simulink model "rc_feedthrough"  (R2025b)
settings: Solver=ode2  StartTime=0.0  StopTime=inf  FixedStep=0.01  RelTol=1e-3
settings Model: Creator=ac112430  LastModifiedBy=ac124458
settings SolverCC: AlgebraicLoopSolver=TrustRegion
settings DataIOCC: ReturnWorkspaceOutputs=off
settings OptimizationCC: DefaultParameterBehavior=Inlined  DefaultUnderspecifiedDataType=single  ReuseModelBlockBuffer=off  PassReuseOutputArgsAs=Individual arguments  EfficientTunableParamExpr=on
settings DebuggingCC: ParameterPrecisionLossMsg=none  ParameterTunabilityLossMsg=error  UnconnectedInputMsg=warning  UnconnectedOutputMsg=warning  UnconnectedLineMsg=warning  ArithmeticOperatorsInVariantConditions=warning
settings HardwareCC: ProdBitPerPointer=32.0  ProdBitPerSizeT=32.0  ProdBitPerPtrDiffT=32.0  ProdLargestAtomicInteger=Long  ProdLargestAtomicFloat=Double  ProdIntDivRoundTo=Undefined  ProdWordSize=32.0  ProdLongLongMode=on  ProdHWDeviceType=ARM Compatible->ARM Cortex
settings ModelReferenceCC: EnableRefExpFcnMdlSchedulingChecks=on  ModelReferenceNumInstancesAllowed=Single  PropagateSignalLabelsOutOfModel=off
settings SFSimCC: SimUseLocalCustomCode=off  MATLABDynamicMemAlloc=off  CustomCodeUndefinedFunction=UseInterfaceOnly
settings RTWCC: SystemTargetFile=ert.tlc  GenCodeOnly=on  TemplateMakefile=ert_default_tmf  RTWUseLocalCustomCode=off  IncludeHyperlinkInReport=on  GPUComputeCapability=3.5  DLArmComputeVersion=19.05  Description=Embedded Coder
settings CodeAppCC: IgnoreCustomStorageClasses=off  MaxIdLength=63.0  StateflowObjectComments=on
settings ERTTargetCC: ERTCustomFileTemplate=example_file_process.tlc  ConvertIfToSwitch=off  SuppressUnreachableDefaultCases=off  DynamicArrayContainerType=coder::array  TargetLangStandard=C99 (ISO)  GenerateSampleERTMain=on  SupportComplex=off

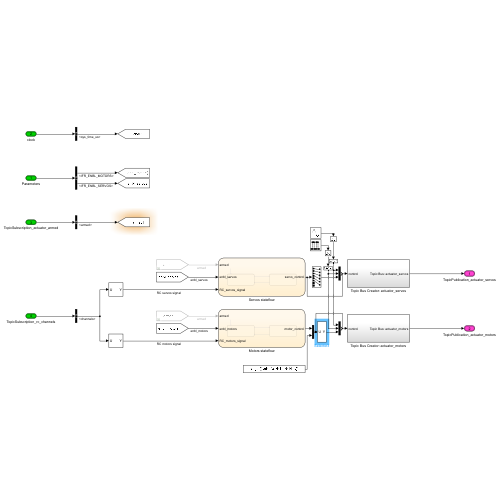
[thumbnail: Simulink's stored preview of the top-level diagram]
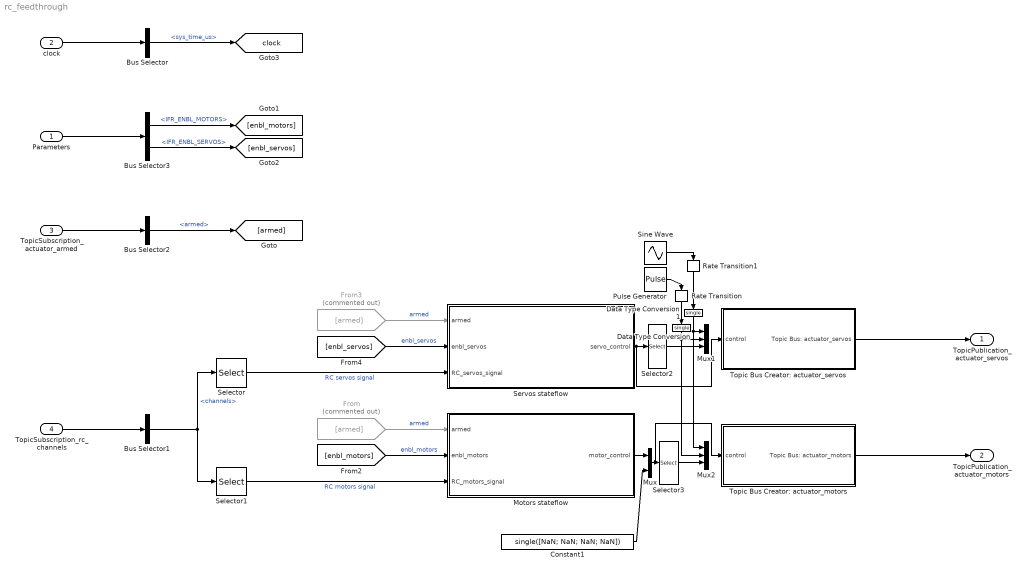
== system rc_feedthrough ==
  Parameters : Inport  OutDataTypeStr=Bus: IFRCG_Bus_Params
  clock : Inport  Port=2  OutDataTypeStr=Bus: IFRCG_Bus_CodeGenInternalClock
  TopicSubscription_actuator_armed : Inport  Port=3  OutDataTypeStr=Bus: IFRCG_Bus_Topic_ActuatorArmed
  TopicSubscription_rc_channels : Inport  Port=4  OutDataTypeStr=Bus: IFRCG_Bus_Topic_RcChannels
  Bus Selector : BusSelector  OutputSignals=sys_time_us
  Bus Selector1 : BusSelector  OutputSignals=channels
  Bus Selector2 : BusSelector  OutputSignals=armed
  Bus Selector3 : BusSelector  OutputSignals=Ifr_Feedthrough.IFR_ENBL_MOTORS,Ifr_Feedthrough.IFR_ENBL_SERVOS
  Constant1 : Constant  Value=single([NaN; NaN; NaN; NaN])  OutDataTypeStr=single
  Data Type Conversion : DataTypeConversion  OutDataTypeStr=single  SaturateOnIntegerOverflow=off  RndMeth=Floor
  Data Type Conversion1 : DataTypeConversion  OutDataTypeStr=single  SaturateOnIntegerOverflow=off  RndMeth=Floor
  From : From  Commented=on  GotoTag=armed
  From3 : From  Commented=on  GotoTag=armed
  Motors stateflow : Stateflow chart  TreatAsAtomicUnit=on
  Mux : Mux  Inputs=2
  Mux1 : Mux  Inputs=3
  Mux2 : Mux  Inputs=3
  Pulse Generator : DiscretePulseGenerator  Period=1000  PulseWidth=50  SampleTime=-1
  Rate Transition : RateTransition
  Rate Transition1 : RateTransition
  Selector : Selector  InputPortWidth=18  IndexOptions=Index vector (dialog)  Indices=[1 2 3 4 5 6 15 16]  OutputSizes=1
  Selector1 : Selector  InputPortWidth=18  IndexOptions=Index vector (dialog)  Indices=[7 8 9 10 11 12 13 14]  OutputSizes=1
  Selector2 : Selector  InputPortWidth=8  IndexOptions=Index vector (dialog)  Indices=1:6  OutputSizes=1
  Selector3 : Selector  InputPortWidth=12  IndexOptions=Index vector (dialog)  Indices=1:10  OutputSizes=1
  Servos stateflow : Stateflow chart  TreatAsAtomicUnit=on
  Sine Wave : Sin  SineType=Sample based  Samples=1000  SampleTime=0.01
  Topic Bus Creator: actuator_motors : Subsystem
  Topic Bus Creator: actuator_servos : Subsystem
  TopicPublication_actuator_servos : Outport  OutDataTypeStr=Bus: IFRCG_Bus_Topic_ActuatorServos  SampleTime=[0.01,0]  VectorParamsAs1DForOutWhenUnconnected=off
  TopicPublication_actuator_motors : Outport  Port=2  OutDataTypeStr=Bus: IFRCG_Bus_Topic_ActuatorMotors  SampleTime=[0.01,0]  VectorParamsAs1DForOutWhenUnconnected=off
  tag scope: clock=global
  wires:
  clock/1 -> Bus Selector/1
  Parameters/1 -> Bus Selector3/1
  Bus Selector3/1 -> [enbl_motors]  "<IFR_ENBL_MOTORS>"
  TopicSubscription_actuator_armed/1 -> Bus Selector2/1
  Bus Selector2/1 -> [armed]  "<armed>"
  TopicSubscription_rc_channels/1 -> Bus Selector1/1
  Bus Selector1/1 -> Selector1/1, Selector/1  "<channels>"
  Selector/1 -> Servos stateflow/3(RC_servos_signal)  "RC servos signal"
  Selector1/1 -> Motors stateflow/3(RC_motors_signal)  "RC motors signal"
  Bus Selector3/2 -> [enbl_servos]  "<IFR_ENBL_SERVOS>"
  From/1 -> Motors stateflow/1(armed)  "armed"
  [enbl_motors] -> Motors stateflow/2(enbl_motors)  "enbl_motors"
  [enbl_servos] -> Servos stateflow/2(enbl_servos)  "enbl_servos"
  From3/1 -> Servos stateflow/1(armed)  "armed"
  Topic Bus Creator: actuator_servos/1(Topic Bus: actuator_servos) -> TopicPublication_actuator_servos/1
  Topic Bus Creator: actuator_motors/1(Topic Bus: actuator_motors) -> TopicPublication_actuator_motors/1
  Constant1/1 -> Mux/2
  Bus Selector/1 -> [clock]  "<sys_time_us>"
  Selector2/1 -> Mux1/3
  Pulse Generator/1 -> Rate Transition/1
  Sine Wave/1 -> Rate Transition1/1
  Servos stateflow/1(servo_control) -> Topic Bus Creator: actuator_servos/1(control), Selector2/1
  Motors stateflow/1(motor_control) -> Mux/1
  Selector3/1 -> Mux2/3
  Rate Transition/1 -> Data Type Conversion/1
  Rate Transition1/1 -> Data Type Conversion1/1
  Data Type Conversion/1 -> Mux1/2, Mux2/2
  Data Type Conversion1/1 -> Mux1/1, Mux2/1
  Mux/1 -> Selector3/1, Topic Bus Creator: actuator_motors/1(control)

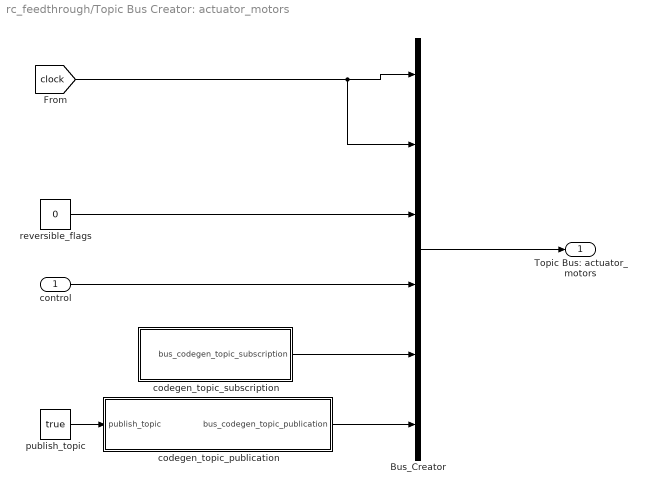
== system rc_feedthrough/Topic Bus Creator: actuator_motors ==
  control : Inport  OutDataTypeStr=single  PortDimensions=12
  Bus_Creator : BusCreator  Inputs=6  OutDataTypeStr=Bus: IFRCG_Bus_Topic_ActuatorMotors
      settings: InheritFromInputs=off
  codegen_topic_publication : Subsystem
  codegen_topic_subscription : Subsystem
  publish_topic : Constant  Value=true  OutDataTypeStr=boolean
  reversible_flags : Constant  Value=0  OutDataTypeStr=uint16
  Topic Bus: actuator_motors : Outport  OutDataTypeStr=Bus: IFRCG_Bus_Topic_ActuatorMotors
  wires:
  Bus_Creator/1 -> Topic Bus: actuator_motors/1
  publish_topic/1 -> codegen_topic_publication/1(publish_topic)
  control/1 -> Bus_Creator/4
  codegen_topic_subscription/1(bus_codegen_topic_subscription) -> Bus_Creator/5
  codegen_topic_publication/1(bus_codegen_topic_publication) -> Bus_Creator/6
  [clock] -> Bus_Creator/2, Bus_Creator/1
  reversible_flags/1 -> Bus_Creator/3

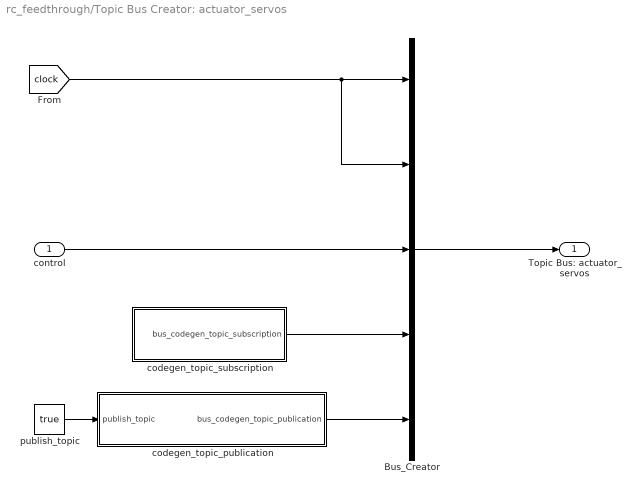
== system rc_feedthrough/Topic Bus Creator: actuator_servos ==
  control : Inport  OutDataTypeStr=single  PortDimensions=8
  Bus_Creator : BusCreator  Inputs=5  OutDataTypeStr=Bus: IFRCG_Bus_Topic_ActuatorServos
      settings: InheritFromInputs=off
  codegen_topic_publication : Subsystem
  codegen_topic_subscription : Subsystem
  publish_topic : Constant  Value=true  OutDataTypeStr=boolean
  Topic Bus: actuator_servos : Outport  OutDataTypeStr=Bus: IFRCG_Bus_Topic_ActuatorServos
  wires:
  Bus_Creator/1 -> Topic Bus: actuator_servos/1
  publish_topic/1 -> codegen_topic_publication/1(publish_topic)
  control/1 -> Bus_Creator/3
  codegen_topic_subscription/1(bus_codegen_topic_subscription) -> Bus_Creator/4
  codegen_topic_publication/1(bus_codegen_topic_publication) -> Bus_Creator/5
  [clock] -> Bus_Creator/2, Bus_Creator/1

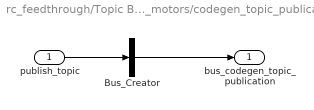
== system rc_feedthrough/Topic Bus Creator: actuator_motors/codegen_topic_publication ==
  publish_topic : Inport  OutDataTypeStr=boolean
  Bus_Creator : BusCreator  Inputs=1  OutDataTypeStr=Bus: IFRCG_Bus_CodeGenInternalTopicPublication
      settings: InheritFromInputs=off
  bus_codegen_topic_publication : Outport  OutDataTypeStr=Bus: IFRCG_Bus_CodeGenInternalTopicPublication
  wires:
  publish_topic/1 -> Bus_Creator/1
  Bus_Creator/1 -> bus_codegen_topic_publication/1

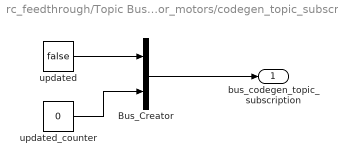
== system rc_feedthrough/Topic Bus Creator: actuator_motors/codegen_topic_subscription ==
  Bus_Creator : BusCreator  Inputs=2  OutDataTypeStr=Bus: IFRCG_Bus_CodeGenInternalTopicSubscription
      settings: InheritFromInputs=off
  updated : Constant  Value=false  OutDataTypeStr=boolean
  updated_counter : Constant  Value=0  OutDataTypeStr=uint64
  bus_codegen_topic_subscription : Outport  OutDataTypeStr=Bus: IFRCG_Bus_CodeGenInternalTopicSubscription
  wires:
  updated_counter/1 -> Bus_Creator/2
  updated/1 -> Bus_Creator/1
  Bus_Creator/1 -> bus_codegen_topic_subscription/1

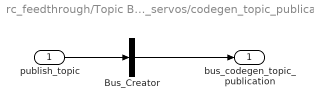
== system rc_feedthrough/Topic Bus Creator: actuator_servos/codegen_topic_publication ==
  publish_topic : Inport  OutDataTypeStr=boolean
  Bus_Creator : BusCreator  Inputs=1  OutDataTypeStr=Bus: IFRCG_Bus_CodeGenInternalTopicPublication
      settings: InheritFromInputs=off
  bus_codegen_topic_publication : Outport  OutDataTypeStr=Bus: IFRCG_Bus_CodeGenInternalTopicPublication
  wires:
  publish_topic/1 -> Bus_Creator/1
  Bus_Creator/1 -> bus_codegen_topic_publication/1

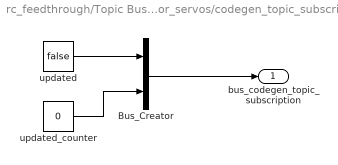
== system rc_feedthrough/Topic Bus Creator: actuator_servos/codegen_topic_subscription ==
  Bus_Creator : BusCreator  Inputs=2  OutDataTypeStr=Bus: IFRCG_Bus_CodeGenInternalTopicSubscription
      settings: InheritFromInputs=off
  updated : Constant  Value=false  OutDataTypeStr=boolean
  updated_counter : Constant  Value=0  OutDataTypeStr=uint64
  bus_codegen_topic_subscription : Outport  OutDataTypeStr=Bus: IFRCG_Bus_CodeGenInternalTopicSubscription
  wires:
  updated_counter/1 -> Bus_Creator/2
  updated/1 -> Bus_Creator/1
  Bus_Creator/1 -> bus_codegen_topic_subscription/1

== stateflow chart rc_feedthrough/Servos stateflow ==
  state Disarmed
    servo_control = single([NaN; NaN; NaN; NaN; NaN; NaN; NaN; NaN]);
  state Armed
    servo_control = single([...
    RC_servos_signal(1); ...
    RC_servos_signal(2); ...
    RC_servos_signal(3); ...
    RC_servos_signal(4); ...
    RC_servos_signal(5); ...
    RC_servos_signal(6); ...
    RC_servos_signal(7); ...
    RC_servos_signal(8); ...
    ]);
  (default) -> Disarmed
  Disarmed -> Armed : [(enbl_servos > 0.5)]
  Armed -> Disarmed : [~(enbl_servos > 0.5)]
  data: armed input boolean; enbl_servos input single; RC_servos_signal input single; servo_control output single

== stateflow chart rc_feedthrough/Motors stateflow ==
  state Disarmed
    motor_control = single([NaN; NaN; NaN; NaN; NaN; NaN; NaN; NaN]);
  state Armed
    motor_control = single([...
    RC_motors_signal(1); ...
    RC_motors_signal(2); ...
    RC_motors_signal(3); ...
    RC_motors_signal(4); ...
    RC_motors_signal(5); ...
    RC_motors_signal(6); ...
    RC_motors_signal(7); ...
    RC_motors_signal(8); ...
    ]);
  (default) -> Disarmed
  Disarmed -> Armed : [(enbl_motors > 0.5)]
  Armed -> Disarmed : [~(enbl_motors > 0.5)]
  data: armed input boolean; enbl_motors input single; RC_motors_signal input single; motor_control output single
